simulink model "combining_test"  (R2021b)
settings: Solver=VariableStepAuto  StartTime=0.0  StopTime=stop_time-1  RelTol=1e-3
libraries: dspsrcs4 x3
settings Model: Creator=torha  LastModifiedBy=torha

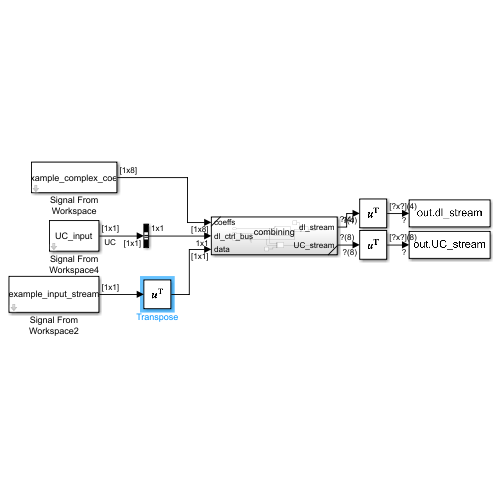
[thumbnail: Simulink's stored preview of the top-level diagram]
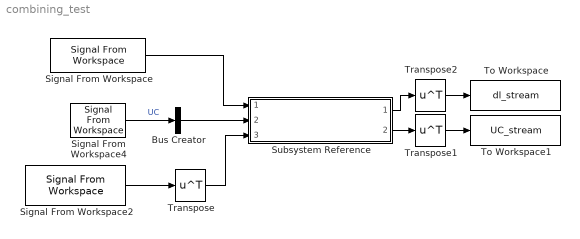
== system combining_test ==
  Bus Creator : BusCreator  Inputs=1
  Signal From Workspace : dspsrcs4/Signal From Workspace  X=example_complex_coeff  Ts=1  nsamps=1  OutputAfterFinalValue=Setting to zero  ignoreOrWarnInputAndFrameLengths=off  OutputFrames=off
  Signal From Workspace2 : dspsrcs4/Signal From Workspace  X=example_input_stream  Ts=1  nsamps=1  OutputAfterFinalValue=Setting to zero  ignoreOrWarnInputAndFrameLengths=off  OutputFrames=off
  Signal From Workspace4 : dspsrcs4/Signal From Workspace  X=UC_input  Ts=1  nsamps=1  OutputAfterFinalValue=Setting to zero  ignoreOrWarnInputAndFrameLengths=off  OutputFrames=off
  Subsystem Reference : Subsystem  ReferencedSubsystem=combining
  To Workspace : ToWorkspace  VariableName=dl_stream  SampleTime=-1
      settings: Save2DSignal=2-D array (concatenate along first dimension)
  To Workspace1 : ToWorkspace  VariableName=UC_stream  SampleTime=-1
      settings: Save2DSignal=2-D array (concatenate along first dimension)
  Transpose : Math  Operator=transpose  SaturateOnIntegerOverflow=on
  Transpose1 : Math  Operator=transpose  SaturateOnIntegerOverflow=on
  Transpose2 : Math  Operator=transpose  SaturateOnIntegerOverflow=on
  wires:
  Signal From Workspace/1 -> Subsystem Reference/1
  Signal From Workspace2/1 -> Transpose/1
  Subsystem Reference/1 -> Transpose2/1
  Bus Creator/1 -> Subsystem Reference/2
  Subsystem Reference/2 -> Transpose1/1
  Signal From Workspace4/1 -> Bus Creator/1  "UC"
  Transpose/1 -> Subsystem Reference/3
  Transpose1/1 -> To Workspace1/1
  Transpose2/1 -> To Workspace/1
